simulink model "IOControls"  (R2019b)
settings: configuration reference "ConfigSet_IOControls_Reference" (kept outside this file)
model workspace (MAT data in the model file):
  SampleTime = 0.05
libraries: IOStateMachinesLib x274, SignalGeneratorsLib x1, simulink x1
(part 10 of 10)

== system IOControls/ForEachVehicle/IOControls/CabControl/DriverDeskLeft/OperatingPanel2/VCBClosePB ==
  note: States:
      | Off
      | On
  InputControl : Inport  OutDataTypeStr=Bus: BD_IOControls_In_InputControl
  Initialise : Inport  Port=2
  Bus Selector : BusSelector  OutputSignals=Value,Mode,InitVal,InternalRequest,Inhibit
  VCBClosePB-Momentary : IOStateMachinesLib/Momentary  InitSource=internal  InitState=InitState
      settings: SourceProductName=IO State Machines
  InputState : Outport  VectorParamsAs1DForOutWhenUnconnected=off
  wires:
  Initialise/1 -> VCBClosePB-Momentary/4
  VCBClosePB-Momentary/1 -> InputState/1
  Bus Selector/5 -> VCBClosePB-Momentary/6  "<Inhibit>"
  Bus Selector/4 -> VCBClosePB-Momentary/5  "<InternalRequest>"
  Bus Selector/3 -> VCBClosePB-Momentary/3  "<InitVal>"
  Bus Selector/2 -> VCBClosePB-Momentary/2  "<Mode>"
  Bus Selector/1 -> VCBClosePB-Momentary/1  "<Value>"
  InputControl/1 -> Bus Selector/1

== system IOControls/ForEachVehicle/IOControls/CabControl/DriverDeskLeft/OperatingPanel2/VCBOpenPB ==
  note: States:
      | Off
      | On
  InputControl : Inport  OutDataTypeStr=Bus: BD_IOControls_In_InputControl
  Initialise : Inport  Port=2
  Bus Selector : BusSelector  OutputSignals=Value,Mode,InitVal,InternalRequest,Inhibit
  VCBOpenPB-Momentary : IOStateMachinesLib/Momentary  InitSource=internal  InitState=InitState
      settings: SourceProductName=IO State Machines
  InputState : Outport  VectorParamsAs1DForOutWhenUnconnected=off
  wires:
  Initialise/1 -> VCBOpenPB-Momentary/4
  VCBOpenPB-Momentary/1 -> InputState/1
  Bus Selector/5 -> VCBOpenPB-Momentary/6  "<Inhibit>"
  Bus Selector/4 -> VCBOpenPB-Momentary/5  "<InternalRequest>"
  Bus Selector/3 -> VCBOpenPB-Momentary/3  "<InitVal>"
  Bus Selector/2 -> VCBOpenPB-Momentary/2  "<Mode>"
  Bus Selector/1 -> VCBOpenPB-Momentary/1  "<Value>"
  InputControl/1 -> Bus Selector/1

== system IOControls/ForEachVehicle/IOControls/CabControl/DriverDeskLeft/OperatingPanel2/WiperPump ==
  note: States:
      | Off
      | On
  InputControl : Inport  OutDataTypeStr=Bus: BD_IOControls_In_InputControl
  Initialise : Inport  Port=2
  Bus Selector : BusSelector  OutputSignals=Value,Mode,InitVal,InternalRequest,Inhibit
  WiperPump-Momentary : IOStateMachinesLib/Momentary  InitSource=internal  InitState=InitState
      settings: SourceProductName=IO State Machines
  InputState : Outport  VectorParamsAs1DForOutWhenUnconnected=off
  wires:
  Initialise/1 -> WiperPump-Momentary/4
  WiperPump-Momentary/1 -> InputState/1
  Bus Selector/5 -> WiperPump-Momentary/6  "<Inhibit>"
  Bus Selector/4 -> WiperPump-Momentary/5  "<InternalRequest>"
  Bus Selector/3 -> WiperPump-Momentary/3  "<InitVal>"
  Bus Selector/2 -> WiperPump-Momentary/2  "<Mode>"
  Bus Selector/1 -> WiperPump-Momentary/1  "<Value>"
  InputControl/1 -> Bus Selector/1

== system IOControls/ForEachVehicle/IOControls/CabControl/DriverDeskLeft/OperatingPanel2/WiperSelectionSwitch ==
  note: States:
      | All
      | Left
      | Middle
      | Right
  InputControl : Inport  OutDataTypeStr=Bus: BD_IOControls_In_InputControl
  Initialise : Inport  Port=2
  Bus Selector : BusSelector  OutputSignals=Value,Mode,InitVal,InternalRequest,Inhibit
  WiperSelectionSwitch-Increment : IOStateMachinesLib/Increment  InitSource=internal  InitState=InitState  ControlStates=ControlStates
      settings: SourceProductName=IO State Machines
  InputState : Outport  VectorParamsAs1DForOutWhenUnconnected=off
  wires:
  Initialise/1 -> WiperSelectionSwitch-Increment/4
  WiperSelectionSwitch-Increment/1 -> InputState/1
  Bus Selector/5 -> WiperSelectionSwitch-Increment/6  "<Inhibit>"
  Bus Selector/4 -> WiperSelectionSwitch-Increment/5  "<InternalRequest>"
  Bus Selector/3 -> WiperSelectionSwitch-Increment/3  "<InitVal>"
  Bus Selector/2 -> WiperSelectionSwitch-Increment/2  "<Mode>"
  Bus Selector/1 -> WiperSelectionSwitch-Increment/1  "<Value>"
  InputControl/1 -> Bus Selector/1

== system IOControls/ForEachVehicle/IOControls/CabControl/DriverDeskRight/OperatingPanel5/BatteryResetPB ==
  note: States:
      | Off
      | On
  InputControl : Inport  OutDataTypeStr=Bus: BD_IOControls_In_InputControl
  Initialise : Inport  Port=2
  BatteryResetPB-Momentary : IOStateMachinesLib/Momentary  InitSource=internal  InitState=InitState
      settings: SourceProductName=IO State Machines
  Bus Selector : BusSelector  OutputSignals=Value,Mode,InitVal,InternalRequest,Inhibit
  InputState : Outport  VectorParamsAs1DForOutWhenUnconnected=off
  wires:
  Initialise/1 -> BatteryResetPB-Momentary/4
  BatteryResetPB-Momentary/1 -> InputState/1
  Bus Selector/5 -> BatteryResetPB-Momentary/6  "<Inhibit>"
  Bus Selector/4 -> BatteryResetPB-Momentary/5  "<InternalRequest>"
  Bus Selector/3 -> BatteryResetPB-Momentary/3  "<InitVal>"
  Bus Selector/2 -> BatteryResetPB-Momentary/2  "<Mode>"
  Bus Selector/1 -> BatteryResetPB-Momentary/1  "<Value>"
  InputControl/1 -> Bus Selector/1

== system IOControls/ForEachVehicle/IOControls/CabControl/DriverDeskRight/OperatingPanel5/CabBoosterFanSS ==
  note: States:
      | Off
      | Low Speed
      | High Speed
  InputControl : Inport  OutDataTypeStr=Bus: BD_IOControls_In_InputControl
  Initialise : Inport  Port=2
  Bus Selector : BusSelector  OutputSignals=Value,Mode,InitVal,InternalRequest,Inhibit
  CabBoosterFanSS-Increment : IOStateMachinesLib/Increment  InitSource=internal  InitState=InitState  ControlStates=ControlStates
      settings: SourceProductName=IO State Machines
  InputState : Outport  VectorParamsAs1DForOutWhenUnconnected=off
  wires:
  Initialise/1 -> CabBoosterFanSS-Increment/4
  CabBoosterFanSS-Increment/1 -> InputState/1
  Bus Selector/5 -> CabBoosterFanSS-Increment/6  "<Inhibit>"
  Bus Selector/4 -> CabBoosterFanSS-Increment/5  "<InternalRequest>"
  Bus Selector/3 -> CabBoosterFanSS-Increment/3  "<InitVal>"
  Bus Selector/2 -> CabBoosterFanSS-Increment/2  "<Mode>"
  Bus Selector/1 -> CabBoosterFanSS-Increment/1  "<Value>"
  InputControl/1 -> Bus Selector/1

== system IOControls/ForEachVehicle/IOControls/CabControl/DriverDeskRight/OperatingPanel5/DoorProvenLoopOutputSwitch ==
  note: States:
      | Normal
      | Cutout
  InputControl : Inport  OutDataTypeStr=Bus: BD_IOControls_In_InputControl
  Initialise : Inport  Port=2
  Bus Selector : BusSelector  OutputSignals=Value,Mode,InitVal,InternalRequest,Inhibit
  DoorProvenLoopOutputSwitch-Toggle : IOStateMachinesLib/Toggle  InitSource=internal  InitState=InitState  OffStateValue=OffStateValue  OnStateValue=OnStateValue
      settings: SourceProductName=IO State Machines
  InputState : Outport  VectorParamsAs1DForOutWhenUnconnected=off
  wires:
  Initialise/1 -> DoorProvenLoopOutputSwitch-Toggle/4
  DoorProvenLoopOutputSwitch-Toggle/1 -> InputState/1
  Bus Selector/5 -> DoorProvenLoopOutputSwitch-Toggle/6  "<Inhibit>"
  Bus Selector/4 -> DoorProvenLoopOutputSwitch-Toggle/5  "<InternalRequest>"
  Bus Selector/3 -> DoorProvenLoopOutputSwitch-Toggle/3  "<InitVal>"
  Bus Selector/2 -> DoorProvenLoopOutputSwitch-Toggle/2  "<Mode>"
  Bus Selector/1 -> DoorProvenLoopOutputSwitch-Toggle/1  "<Value>"
  InputControl/1 -> Bus Selector/1

== system IOControls/ForEachVehicle/IOControls/CabControl/DriverDeskRight/OperatingPanel5/EmergencyBrakePBBypassSS ==
  note: States:
      | Normal
      | Bypass
  InputControl : Inport  OutDataTypeStr=Bus: BD_IOControls_In_InputControl
  Initialise : Inport  Port=2
  Bus Selector : BusSelector  OutputSignals=Value,Mode,InitVal,InternalRequest,Inhibit
  EmergencyBrakePBBypassSS-Toggle : IOStateMachinesLib/Toggle  InitSource=internal  InitState=InitState  OffStateValue=OffStateValue  OnStateValue=OnStateValue
      settings: SourceProductName=IO State Machines
  InputState : Outport  VectorParamsAs1DForOutWhenUnconnected=off
  wires:
  Initialise/1 -> EmergencyBrakePBBypassSS-Toggle/4
  EmergencyBrakePBBypassSS-Toggle/1 -> InputState/1
  Bus Selector/5 -> EmergencyBrakePBBypassSS-Toggle/6  "<Inhibit>"
  Bus Selector/4 -> EmergencyBrakePBBypassSS-Toggle/5  "<InternalRequest>"
  Bus Selector/3 -> EmergencyBrakePBBypassSS-Toggle/3  "<InitVal>"
  Bus Selector/2 -> EmergencyBrakePBBypassSS-Toggle/2  "<Mode>"
  Bus Selector/1 -> EmergencyBrakePBBypassSS-Toggle/1  "<Value>"
  InputControl/1 -> Bus Selector/1

== system IOControls/ForEachVehicle/IOControls/CabControl/DriverDeskRight/OperatingPanel5/EmergencyStopPB ==
  note: States:
      | Off
      | On
  InputControl : Inport  OutDataTypeStr=Bus: BD_IOControls_In_InputControl
  Initialise : Inport  Port=2
  Bus Selector : BusSelector  OutputSignals=Value,Mode,InitVal,InternalRequest,Inhibit
  EmergencyStopPB-Toggle : IOStateMachinesLib/Toggle  InitSource=internal  InitState=InitState  OffStateValue=OffStateValue  OnStateValue=OnStateValue
      settings: SourceProductName=IO State Machines
  InputState : Outport  VectorParamsAs1DForOutWhenUnconnected=off
  wires:
  Initialise/1 -> EmergencyStopPB-Toggle/4
  EmergencyStopPB-Toggle/1 -> InputState/1
  Bus Selector/5 -> EmergencyStopPB-Toggle/6  "<Inhibit>"
  Bus Selector/4 -> EmergencyStopPB-Toggle/5  "<InternalRequest>"
  Bus Selector/3 -> EmergencyStopPB-Toggle/3  "<InitVal>"
  Bus Selector/2 -> EmergencyStopPB-Toggle/2  "<Mode>"
  Bus Selector/1 -> EmergencyStopPB-Toggle/1  "<Value>"
  InputControl/1 -> Bus Selector/1

== system IOControls/ForEachVehicle/IOControls/CabControl/DriverDeskRight/OperatingPanel5/FlasherLightPB ==
  note: States:
      | Off
      | On
  InputControl : Inport  OutDataTypeStr=Bus: BD_IOControls_In_InputControl
  Initialise : Inport  Port=2
  Bus Selector : BusSelector  OutputSignals=Value,Mode,InitVal,InternalRequest,Inhibit
  FlasherLightPB-Toggle : IOStateMachinesLib/Toggle  InitSource=internal  InitState=InitState  OffStateValue=OffStateValue  OnStateValue=OnStateValue
      settings: SourceProductName=IO State Machines
  InputState : Outport  VectorParamsAs1DForOutWhenUnconnected=off
  wires:
  Initialise/1 -> FlasherLightPB-Toggle/4
  FlasherLightPB-Toggle/1 -> InputState/1
  Bus Selector/5 -> FlasherLightPB-Toggle/6  "<Inhibit>"
  Bus Selector/4 -> FlasherLightPB-Toggle/5  "<InternalRequest>"
  Bus Selector/3 -> FlasherLightPB-Toggle/3  "<InitVal>"
  Bus Selector/2 -> FlasherLightPB-Toggle/2  "<Mode>"
  Bus Selector/1 -> FlasherLightPB-Toggle/1  "<Value>"
  InputControl/1 -> Bus Selector/1

== system IOControls/ForEachVehicle/IOControls/CabControl/DriverDeskRight/OperatingPanel5/FloodLightPB ==
  note: States:
      | Off
      | On
  InputControl : Inport  OutDataTypeStr=Bus: BD_IOControls_In_InputControl
  Initialise : Inport  Port=2
  Bus Selector : BusSelector  OutputSignals=Value,Mode,InitVal,InternalRequest,Inhibit
  FloodLightPB-Toggle : IOStateMachinesLib/Toggle  InitSource=internal  InitState=InitState  OffStateValue=OffStateValue  OnStateValue=OnStateValue
      settings: SourceProductName=IO State Machines
  InputState : Outport  VectorParamsAs1DForOutWhenUnconnected=off
  wires:
  Initialise/1 -> FloodLightPB-Toggle/4
  FloodLightPB-Toggle/1 -> InputState/1
  Bus Selector/5 -> FloodLightPB-Toggle/6  "<Inhibit>"
  Bus Selector/4 -> FloodLightPB-Toggle/5  "<InternalRequest>"
  Bus Selector/3 -> FloodLightPB-Toggle/3  "<InitVal>"
  Bus Selector/2 -> FloodLightPB-Toggle/2  "<Mode>"
  Bus Selector/1 -> FloodLightPB-Toggle/1  "<Value>"
  InputControl/1 -> Bus Selector/1

== system IOControls/ForEachVehicle/IOControls/CabControl/DriverDeskRight/OperatingPanel5/HoldDoorCloseBypassSS ==
  note: States:
      | Normal
      | HDCB Left
      | HDCB Right
  InputControl : Inport  OutDataTypeStr=Bus: BD_IOControls_In_InputControl
  Initialise : Inport  Port=2
  Bus Selector : BusSelector  OutputSignals=Value,Mode,InitVal,InternalRequest,Inhibit
  HoldDoorCloseBypassSS-Increment : IOStateMachinesLib/Increment  InitSource=internal  InitState=InitState  ControlStates=ControlStates
      settings: SourceProductName=IO State Machines
  InputState : Outport  VectorParamsAs1DForOutWhenUnconnected=off
  wires:
  Initialise/1 -> HoldDoorCloseBypassSS-Increment/4
  HoldDoorCloseBypassSS-Increment/1 -> InputState/1
  Bus Selector/5 -> HoldDoorCloseBypassSS-Increment/6  "<Inhibit>"
  Bus Selector/4 -> HoldDoorCloseBypassSS-Increment/5  "<InternalRequest>"
  Bus Selector/3 -> HoldDoorCloseBypassSS-Increment/3  "<InitVal>"
  Bus Selector/2 -> HoldDoorCloseBypassSS-Increment/2  "<Mode>"
  Bus Selector/1 -> HoldDoorCloseBypassSS-Increment/1  "<Value>"
  InputControl/1 -> Bus Selector/1

== system IOControls/ForEachVehicle/IOControls/CabControl/DriverDeskRight/OperatingPanel5/LampTestPB ==
  note: States:
      | Off
      | On
  InputControl : Inport  OutDataTypeStr=Bus: BD_IOControls_In_InputControl
  Initialise : Inport  Port=2
  Bus Selector : BusSelector  OutputSignals=Value,Mode,InitVal,InternalRequest,Inhibit
  LampTestPB-Toggle : IOStateMachinesLib/Toggle  InitSource=internal  InitState=InitState  OffStateValue=OffStateValue  OnStateValue=OnStateValue
      settings: SourceProductName=IO State Machines
  InputState : Outport  VectorParamsAs1DForOutWhenUnconnected=off
  wires:
  Initialise/1 -> LampTestPB-Toggle/4
  LampTestPB-Toggle/1 -> InputState/1
  Bus Selector/5 -> LampTestPB-Toggle/6  "<Inhibit>"
  Bus Selector/4 -> LampTestPB-Toggle/5  "<InternalRequest>"
  Bus Selector/3 -> LampTestPB-Toggle/3  "<InitVal>"
  Bus Selector/2 -> LampTestPB-Toggle/2  "<Mode>"
  Bus Selector/1 -> LampTestPB-Toggle/1  "<Value>"
  InputControl/1 -> Bus Selector/1

== system IOControls/ForEachVehicle/IOControls/CabControl/DriverDeskRight/OperatingPanel5/RightDoorClosePBOperatingPanel5 ==
  note: States:
      | Off
      | On
  InputControl : Inport  OutDataTypeStr=Bus: BD_IOControls_In_InputControl
  Initialise : Inport  Port=2
  Bus Selector : BusSelector  OutputSignals=Value,Mode,InitVal,InternalRequest,Inhibit
  RightDoorClosePBOperatingPanel5-Momentary : IOStateMachinesLib/Momentary  InitSource=internal  InitState=InitState
      settings: SourceProductName=IO State Machines
  InputState : Outport  VectorParamsAs1DForOutWhenUnconnected=off
  wires:
  Initialise/1 -> RightDoorClosePBOperatingPanel5-Momentary/4
  RightDoorClosePBOperatingPanel5-Momentary/1 -> InputState/1
  Bus Selector/5 -> RightDoorClosePBOperatingPanel5-Momentary/6  "<Inhibit>"
  Bus Selector/4 -> RightDoorClosePBOperatingPanel5-Momentary/5  "<InternalRequest>"
  Bus Selector/3 -> RightDoorClosePBOperatingPanel5-Momentary/3  "<InitVal>"
  Bus Selector/2 -> RightDoorClosePBOperatingPanel5-Momentary/2  "<Mode>"
  Bus Selector/1 -> RightDoorClosePBOperatingPanel5-Momentary/1  "<Value>"
  InputControl/1 -> Bus Selector/1

== system IOControls/ForEachVehicle/IOControls/CabControl/DriverDeskRight/OperatingPanel5/RightDoorOpenPB1OperatingPanel5 ==
  note: States:
      | Off
      | On
  InputControl : Inport  OutDataTypeStr=Bus: BD_IOControls_In_InputControl
  Initialise : Inport  Port=2
  Bus Selector : BusSelector  OutputSignals=Value,Mode,InitVal,InternalRequest,Inhibit
  RightDoorOpenPB1OperatingPanel5-Momentary : IOStateMachinesLib/Momentary  InitSource=internal  InitState=InitState
      settings: SourceProductName=IO State Machines
  InputState : Outport  VectorParamsAs1DForOutWhenUnconnected=off
  wires:
  Initialise/1 -> RightDoorOpenPB1OperatingPanel5-Momentary/4
  RightDoorOpenPB1OperatingPanel5-Momentary/1 -> InputState/1
  Bus Selector/5 -> RightDoorOpenPB1OperatingPanel5-Momentary/6  "<Inhibit>"
  Bus Selector/4 -> RightDoorOpenPB1OperatingPanel5-Momentary/5  "<InternalRequest>"
  Bus Selector/3 -> RightDoorOpenPB1OperatingPanel5-Momentary/3  "<InitVal>"
  Bus Selector/2 -> RightDoorOpenPB1OperatingPanel5-Momentary/2  "<Mode>"
  Bus Selector/1 -> RightDoorOpenPB1OperatingPanel5-Momentary/1  "<Value>"
  InputControl/1 -> Bus Selector/1

== system IOControls/ForEachVehicle/IOControls/CabControl/DriverDeskRight/OperatingPanel5/RightDoorOpenPBOperatingPanel5 ==
  note: States:
      | Off
      | On
  InputControl : Inport  OutDataTypeStr=Bus: BD_IOControls_In_InputControl
  Initialise : Inport  Port=2
  Bus Selector : BusSelector  OutputSignals=Value,Mode,InitVal,InternalRequest,Inhibit
  RightDoorOpenPBOperatingPanel5-Momentary : IOStateMachinesLib/Momentary  InitSource=internal  InitState=InitState
      settings: SourceProductName=IO State Machines
  InputState : Outport  VectorParamsAs1DForOutWhenUnconnected=off
  wires:
  Initialise/1 -> RightDoorOpenPBOperatingPanel5-Momentary/4
  RightDoorOpenPBOperatingPanel5-Momentary/1 -> InputState/1
  Bus Selector/5 -> RightDoorOpenPBOperatingPanel5-Momentary/6  "<Inhibit>"
  Bus Selector/4 -> RightDoorOpenPBOperatingPanel5-Momentary/5  "<InternalRequest>"
  Bus Selector/3 -> RightDoorOpenPBOperatingPanel5-Momentary/3  "<InitVal>"
  Bus Selector/2 -> RightDoorOpenPBOperatingPanel5-Momentary/2  "<Mode>"
  Bus Selector/1 -> RightDoorOpenPBOperatingPanel5-Momentary/1  "<Value>"
  InputControl/1 -> Bus Selector/1

== system IOControls/ForEachVehicle/IOControls/CabControl/DriverDeskRight/OperatingPanel5/UncouplePB ==
  note: States:
      | Off
      | On
  InputControl : Inport  OutDataTypeStr=Bus: BD_IOControls_In_InputControl
  Initialise : Inport  Port=2
  Bus Selector : BusSelector  OutputSignals=Value,Mode,InitVal,InternalRequest,Inhibit
  UncouplePB-Momentary : IOStateMachinesLib/Momentary  InitSource=internal  InitState=InitState
      settings: SourceProductName=IO State Machines
  InputState : Outport  VectorParamsAs1DForOutWhenUnconnected=off
  wires:
  Initialise/1 -> UncouplePB-Momentary/4
  UncouplePB-Momentary/1 -> InputState/1
  Bus Selector/5 -> UncouplePB-Momentary/6  "<Inhibit>"
  Bus Selector/4 -> UncouplePB-Momentary/5  "<InternalRequest>"
  Bus Selector/3 -> UncouplePB-Momentary/3  "<InitVal>"
  Bus Selector/2 -> UncouplePB-Momentary/2  "<Mode>"
  Bus Selector/1 -> UncouplePB-Momentary/1  "<Value>"
  InputControl/1 -> Bus Selector/1

== system IOControls/ForEachVehicle/IOControls/CabControl/DriverDeskRight/OperatingPanel5/WFLTestPB ==
  note: States:
      | Off
      | On
  InputControl : Inport  OutDataTypeStr=Bus: BD_IOControls_In_InputControl
  Initialise : Inport  Port=2
  Bus Selector : BusSelector  OutputSignals=Value,Mode,InitVal,InternalRequest,Inhibit
  WFLTestPB-Toggle : IOStateMachinesLib/Toggle  InitSource=internal  InitState=InitState  OffStateValue=OffStateValue  OnStateValue=OnStateValue
      settings: SourceProductName=IO State Machines
  InputState : Outport  VectorParamsAs1DForOutWhenUnconnected=off
  wires:
  Initialise/1 -> WFLTestPB-Toggle/4
  WFLTestPB-Toggle/1 -> InputState/1
  Bus Selector/5 -> WFLTestPB-Toggle/6  "<Inhibit>"
  Bus Selector/4 -> WFLTestPB-Toggle/5  "<InternalRequest>"
  Bus Selector/3 -> WFLTestPB-Toggle/3  "<InitVal>"
  Bus Selector/2 -> WFLTestPB-Toggle/2  "<Mode>"
  Bus Selector/1 -> WFLTestPB-Toggle/1  "<Value>"
  InputControl/1 -> Bus Selector/1

== system IOControls/ForEachVehicle/IOControls/CabControl/DriverDeskRight/OperatingPanel5/WiperControlSwitch ==
  note: States:
      |
      | Park
      | Off
      | Low Speed
      | High Speed
  InputControl : Inport  OutDataTypeStr=Bus: BD_IOControls_In_InputControl
  Initialise : Inport  Port=2
  Bus Selector : BusSelector  OutputSignals=Value,Mode,InitVal,InternalRequest,Inhibit
  WiperControlSwitch-Increment : IOStateMachinesLib/Increment  InitSource=internal  InitState=InitState  ControlStates=ControlStates
      settings: SourceProductName=IO State Machines
  InputState : Outport  VectorParamsAs1DForOutWhenUnconnected=off
  wires:
  Initialise/1 -> WiperControlSwitch-Increment/4
  WiperControlSwitch-Increment/1 -> InputState/1
  Bus Selector/5 -> WiperControlSwitch-Increment/6  "<Inhibit>"
  Bus Selector/4 -> WiperControlSwitch-Increment/5  "<InternalRequest>"
  Bus Selector/3 -> WiperControlSwitch-Increment/3  "<InitVal>"
  Bus Selector/2 -> WiperControlSwitch-Increment/2  "<Mode>"
  Bus Selector/1 -> WiperControlSwitch-Increment/1  "<Value>"
  InputControl/1 -> Bus Selector/1
